simulink subsystem "flightModeSystem"  (R2026a)
settings: Solver=VariableStepAuto
settings Model: Creator=maxhu  LastModifiedBy=maxhu

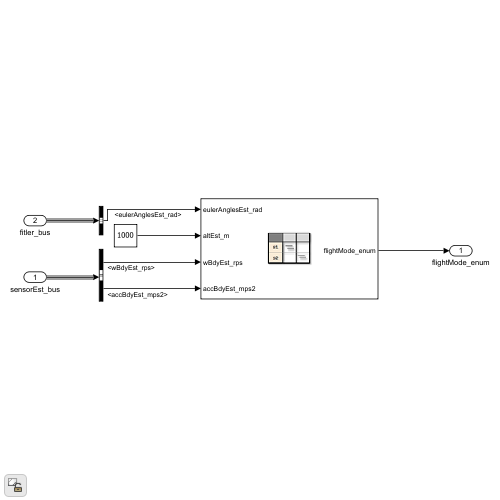
[thumbnail: Simulink's stored preview of the top-level diagram]
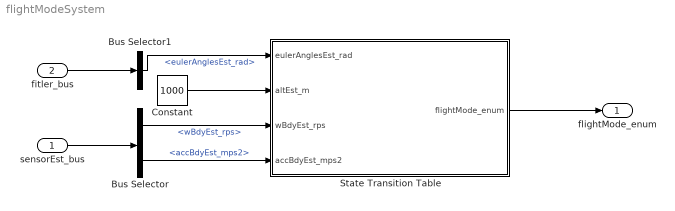
== system flightModeSystem ==
  sensorEst_bus : Inport
  fitler_bus : Inport  Port=2
  Bus Selector : BusSelector  OutputSignals=wBdyEst_rps,accBdyEst_mps2
  Bus Selector1 : BusSelector  OutputSignals=eulerAnglesEst_rad
  Constant : Constant  Value=1000
  State Transition Table : State Transition Table  TreatAsAtomicUnit=on
  flightMode_enum : Outport
  wires:
  sensorEst_bus/1 -> Bus Selector/1
  Bus Selector/2 -> State Transition Table/4(accBdyEst_mps2)  "<accBdyEst_mps2>"
  Bus Selector/1 -> State Transition Table/3(wBdyEst_rps)  "<wBdyEst_rps>"
  State Transition Table/1(flightMode_enum) -> flightMode_enum/1
  Constant/1 -> State Transition Table/2(altEst_m)
  Bus Selector1/1 -> State Transition Table/1(eulerAnglesEst_rad)  "<eulerAnglesEst_rad>"
  fitler_bus/1 -> Bus Selector1/1

== stateflow chart flightModeSystem/State Transition Table ==
  state Idle
    entry:
    flightMode_enum = flightMode.IDLE;
    boostThreshold_b = false;
    during:
    boostThreshold_b = norm(accBdyEst_mps2) > navStates.boostThreshold_mps2;
  state Boost
    entry:
    flightMode_enum = flightMode.BOOST;
    coastThreshold_b = false;
    during:
    coastThreshold_b = altEst_m > navStates.coastThresholdAlt_m && ...
    accBdyEst_mps2(1) < navStates.coastThresholdxAcc_mps2;
  state PastCoastThreshold
    during:
    coastThreshold_b = altEst_m > navStates.coastThresholdAlt_m && ...
    accBdyEst_mps2(1) < navStates.coastThresholdxAcc_mps2;
  state Active
    entry:
    flightMode_enum = flightMode.ACTIVE;
    lockoutThreshold_b = false;
    during:
    lockoutThreshold_b = wBdyEst_rps(2) > navStates.controlTresholdPitchYawRate_rps || ...
    wBdyEst_rps(3) > navStates.controlTresholdPitchYawRate_rps || ...
    eulerAnglesEst_rad(2) > navStates.controlTresholdPitchYaw_rad || ...
    eulerAnglesEst_rad(3) > navStates.controlTresholdPitchYaw_rad;
  state PastLockoutThreshold
    during:
    lockoutThreshold_b = wBdyEst_rps(2) > navStates.controlTresholdPitchYawRate_rps || ...
    wBdyEst_rps(3) > navStates.controlTresholdPitchYawRate_rps || ...
    eulerAnglesEst_rad(2) > navStates.controlTresholdPitchYaw_rad || ...
    eulerAnglesEst_rad(3) > navStates.controlTresholdPitchYaw_rad;
  state Lockout
    entry:
    flightMode_enum = flightMode.LOCKOUT;
  (default) -> Idle
  Idle -> Boost : [boostThreshold_b]
  Boost -> PastCoastThreshold : [coastThreshold_b]
  PastCoastThreshold -> Boost [order 1] : [~coastThreshold_b]
  PastCoastThreshold -> Active [order 2] : [elapsed(sec) > navStates.debounce_s]
  Active -> PastLockoutThreshold : [lockoutThreshold_b]
  PastLockoutThreshold -> Active [order 1] : [~lockoutThreshold_b]
  PastLockoutThreshold -> Lockout [order 2] : [elapsed(sec) > navStates.debounce_s]
  data: eulerAnglesEst_rad input; boostThreshold_b local; lockoutThreshold_b local; flightMode_enum output; altEst_m input; coastThreshold_b local; wBdyEst_rps input; accBdyEst_mps2 input; navStates parameter
